simulink model "DCmotorSimulink_Torque_control"  (R2023b)
settings: Solver=VariableStepAuto  StartTime=0.0  StopTime=0.05  RelTol=1e-3
values from neighbouring files (symbols this model uses):
  i_a_rated = 27    [DCmotor_Torque_control_parameters.m]
  J = 0.068    [DCmotor_Torque_control_parameters.m]
  Ka = 1    [DCmotor_Torque_control_parameters.m]
  La = 2.3e-3    (= 0.0023)    [DCmotor_Torque_control_parameters.m]
  M = 1.304    [DCmotor_Torque_control_parameters.m]
  R_f = 356.7    [DCmotor_Torque_control_parameters.m]
  Ra = 0.3    [DCmotor_Torque_control_parameters.m]
  Tload = 10    [DCmotor_Torque_control_parameters.m]
  Tref = 10    [DCmotor_Torque_control_parameters.m]
  v_f = 240    [DCmotor_Torque_control_parameters.m]
  v_t_rated = 230    [DCmotor_Torque_control_parameters.m]
libraries: slpidlib x1
settings Model: Creator=chayutht  LastModifiedBy=chayutht

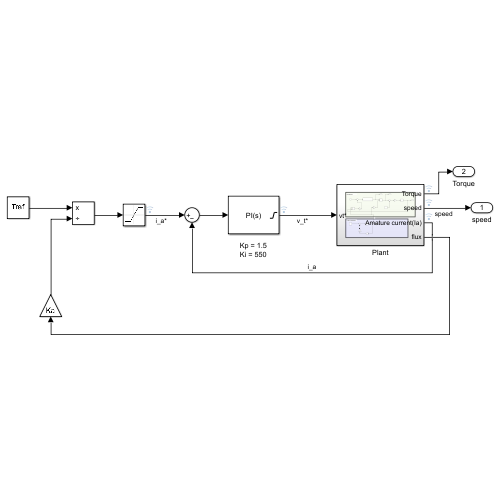
[thumbnail: Simulink's stored preview of the top-level diagram]
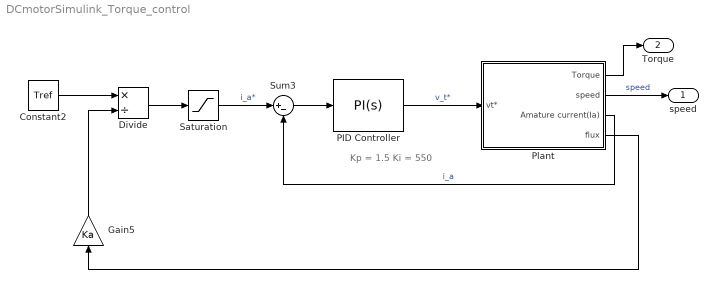
== system DCmotorSimulink_Torque_control ==
  note: Kp = 1.5
      | Ki = 550
  Constant2 : Constant  Value=Tref
  Divide : Product  Inputs=*/
  Gain5 : Gain  Gain=Ka
  PID Controller : slpidlib/PID Controller  Controller=PI  Form=Parallel  TimeDomain=Continuous-time  UseExternalTs=off  SampleTime=-1  IntegratorMethod=Forward Euler  FilterMethod=Forward Euler  ControllerParametersSource=internal  P=1.5  I=550  UseKiTs=off  D=0  N=100  UseFilter=on  TunerSelectOption=Transfer Function Based (PID Tuner App)  InitialConditionSource=internal  InitialConditionForIntegrator=0  InitialConditionForFilter=0  DifferentiatorICPrevScaledInput=0  ExternalReset=none  TrackingMode=off  Kt=1  LimitOutput=on  SatLimitsSource=internal  UpperSaturationLimit=v_t_rated  LowerSaturationLimit=-v_t_rated  LinearizeAsGain=on  AntiWindupMode=none  Kb=1  LimitIntegrator=off  UpperIntegratorSaturationLimit=inf  LowerIntegratorSaturationLimit=-inf  POutMin=[]  POutMax=[]  IOutMin=[]  IOutMax=[]  DOutMin=[]  DOutMax=[]  NOutMin=[]  NOutMax=[]  SumOutMin=[]  SumOutMax=[]  SaturationOutMin=[]  SaturationOutMax=[]  PParamMin=[]  PParamMax=[]  IParamMin=[]  IParamMax=[]  DParamMin=[]  DParamMax=[]  NParamMin=[]  NParamMax=[]  KbParamMin=[]  KbParamMax=[]  KtParamMin=[]  KtParamMax=[]  KbOutMin=[]  KbOutMax=[]  KtOutMin=[]  KtOutMax=[]  IntegratorOutMin=[]  IntegratorOutMax=[]  FilterOutMin=[]  FilterOutMax=[]  SumI1OutMin=[]  SumI1OutMax=[]  SumI2OutMin=[]  SumI2OutMax=[]  SumI3OutMin=[]  SumI3OutMax=[]  SumI4OutMin=[]  SumI4OutMax=[]  SumDOutMin=[]  SumDOutMax=[]  DifferentiatorOutMin=[]  DifferentiatorOutMax=[]  FilterDiffOutCoefMin=[]  FilterDiffOutCoefMax=[]  ReciprocalOutMin=[]  ReciprocalOutMax=[]  SumDenOutMin=[]  SumDenOutMax=[]  SumNumOutMin=[]  SumNumOutMax=[]  DivideOutMin=[]  DivideOutMax=[]  UdiffTsProdOutMin=[]  UdiffTsProdOutMax=[]  NTsProdOutMin=[]  NTsProdOutMax=[]  UintegralTsProdOutMin=[]  UintegralTsProdOutMax=[]  UngainTsProdOutMin=[]  UngainTsProdOutMax=[]  ClampingZeroOutDataTypeStr=Inherit: Inherit via back propagation  ClampingZeroOutMin=[]  ClampingZeroOutMax=[]  FilterDenConstantOutDataTypeStr=Inherit: Inherit via back propagation  FilterDenConstantOutMin=[]  FilterDenConstantOutMax=[]  PCopyOutDataTypeStr=Inherit: Inherit via back propagation  PCopyOutMin=[]  PCopyOutMax=[]  NCopyOutDataTypeStr=Inherit: Inherit via back propagation  NCopyOutMin=[]  NCopyOutMax=[]  IntegratorContinuousStateAttributes=''  IntegratorStateMustResolveToSignalObject=off  IntegratorRTWStateStorageClass=Auto  FilterContinuousStateAttributes=''  FilterStateMustResolveToSignalObject=off  FilterRTWStateStorageClass=Auto  ParallelPVariant=InternalParameters  IdealPVariant=Disabled  IVariant=InternalParameters  DVariant=Disabled  IntegratorVariant=Continuous  SatVariant=Enabled  AWVariant=Passthrough  PCopyVariant=Disabled  TRVariant=Disabled  FdbkBlocksVariant=Forward  IdealPFdbkVariant=Disabled  SatFdbkVariant=Disabled  DerivativeFilterVariant=Disabled  NVariant=Disabled  NCopyVariant=Disabled_SignalSpec  FilterICVariant=Disabled  IntegratorICVariant=InternalICs  ExternalResetVariant=Disabled  TRSumVariant=Passthrough  SumFdbkVariant=Disabled  SumVariant=Sum_PI  TsampFilterVariant=InternalTs  TsampNgainVariant=Passthrough  TsampIntegralVariant=Disabled_SignalSpec  ExternalSaturationOutDataTypeStr=Inherit: Same as second input
  Plant : Subsystem
  Saturation : Saturate  UpperLimit=i_a_rated  LowerLimit=-i_a_rated
  Sum3 : Sum  Inputs=|+-
  speed : Outport
  Torque : Outport  Port=2
  wires:
  Sum3/1 -> PID Controller/1
  Constant2/1 -> Divide/1
  Divide/1 -> Saturation/1
  Gain5/1 -> Divide/2
  PID Controller/1 -> Plant/1(vt*)  "v_t*"
  Plant/1(Torque) -> Torque/1
  Plant/2(speed) -> speed/1  "speed"
  Plant/3(Amature current(Ia)) -> Sum3/2  "i_a"
  Plant/4(flux) -> Gain5/1
  Saturation/1 -> Sum3/1  "i_a*"

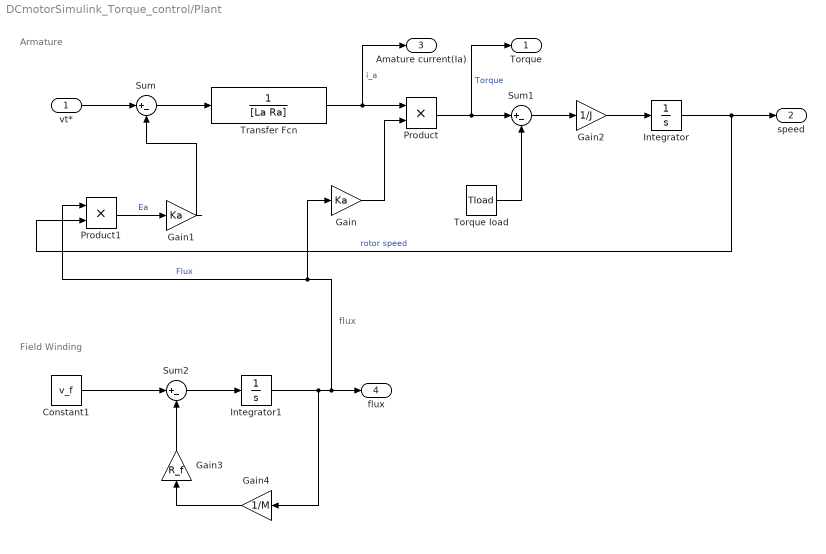
== system DCmotorSimulink_Torque_control/Plant ==
  note: flux
  note: Armature
  note: Field Winding
  vt* : Inport
  Constant1 : Constant  Value=v_f
  Gain : Gain  Gain=Ka
  Gain1 : Gain  Gain=Ka
  Gain2 : Gain  Gain=1/J
  Gain3 : Gain  Gain=R_f
  Gain4 : Gain  Gain=1/M
  Integrator : Integrator
  Integrator1 : Integrator  InitialCondition=0.8476
  Product : Product
  Product1 : Product
  Sum : Sum  Inputs=|+-
  Sum1 : Sum  Inputs=|+-
  Sum2 : Sum  Inputs=|+-
  Torque load : Constant  Value=Tload
  Transfer Fcn : TransferFcn  Denominator=[La Ra]
      settings: AttributesFormatString=%<Denominator>=(0.0023 0.3)
  Torque : Outport
  speed : Outport  Port=2
  Amature current(Ia) : Outport  Port=3
  flux : Outport  Port=4
  wires:
  Gain/1 -> Product/2
  Integrator/1 -> Product1/2, speed/1  "rotor speed"
  Torque load/1 -> Sum1/2
  Integrator1/1 -> Product1/1, Gain/1, flux/1, Gain4/1  "Flux"
  Sum1/1 -> Gain2/1
  vt*/1 -> Sum/1
  Product/1 -> Torque/1, Sum1/1  "Torque"
  Gain2/1 -> Integrator/1
  Gain3/1 -> Sum2/2
  Gain1/1 -> Sum/2
  Product1/1 -> Gain1/1  "Ea"
  Gain4/1 -> Gain3/1
  Transfer Fcn/1 -> Product/1, Amature current(Ia)/1  "i_a"
  Sum2/1 -> Integrator1/1
  Sum/1 -> Transfer Fcn/1
  Constant1/1 -> Sum2/1
